simulink library "controllerComponents"  (R2018a)
settings: Solver=VariableStepAuto  StartTime=0.0  StopTime=10.0  RelTol=1e-3
undefined symbols (not defined in the file): p
libraries: simulink x2, dspsigops x1
settings Model: Creator=mitch  LastModifiedBy=mcobb

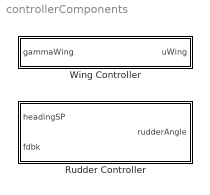
== system controllerComponents ==
  Rudder Controller : Subsystem
  Wing Controller : Subsystem

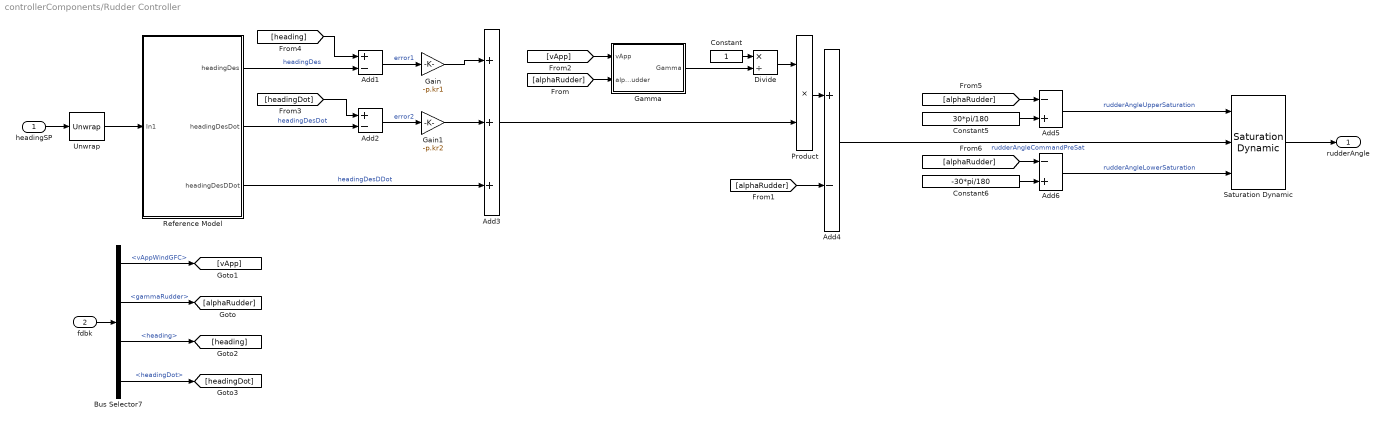
== system controllerComponents/Rudder Controller ==
  headingSP : Inport  Unit=rad
  fdbk : Inport  Port=2  OutDataTypeStr=Bus: busPlantFeedback
  Add1 : Sum  Inputs=+-
  Add2 : Sum  Inputs=+-
  Add3 : Sum  Inputs=+++
  Add4 : Sum  Inputs=+-
  Add5 : Sum  Inputs=-+
  Add6 : Sum  Inputs=-+
  Bus Selector7 : BusSelector  OutputSignals=vAppWindGFC,gammaRudder,heading,headingDot
  Constant : Constant
  Constant5 : Constant  Value=30*pi/180
  Constant6 : Constant  Value=-30*pi/180
  Divide : Product  Inputs=*/
  Gain : Gain  Gain=-p.kr1
  Gain1 : Gain  Gain=-p.kr2
  Gamma : Subsystem
  Product : Product
  Reference Model : Subsystem
  Saturation Dynamic : simulink/Discontinuities/Saturation Dynamic  OutMin=[]  OutMax=[]  OutDataTypeStr=Inherit: Same as second input  OutDataType=fixdt(1, 16)  OutScaling=2^-10  DoSatur=off
  Unwrap : dspsigops/Unwrap  tol=pi  InputProcessing=Columns as channels (frame based)  running=off
  rudderAngle : Outport  Unit=rad
  wires:
  [vApp] -> Gamma/1(vApp)
  [alphaRudder] -> Gamma/2(alphaRudder)
  [alphaRudder] -> Add4/2
  Product/1 -> Add4/1
  Gamma/1(Gamma) -> Divide/2
  Divide/1 -> Product/1
  Constant/1 -> Divide/1
  Add2/1 -> Gain1/1  "error2"
  Add1/1 -> Gain/1  "error1"
  Reference Model/1(headingDes) -> Add1/2  "headingDes"
  Reference Model/2(headingDesDot) -> Add2/2  "headingDesDot"
  [heading] -> Add1/1
  Gain1/1 -> Add3/2
  [headingDot] -> Add2/1
  Reference Model/3(headingDesDDot) -> Add3/3  "headingDesDDot"
  Gain/1 -> Add3/1
  Add3/1 -> Product/2
  fdbk/1 -> Bus Selector7/1
  Bus Selector7/4 -> [headingDot]  "<headingDot>"
  Bus Selector7/3 -> [heading]  "<heading>"
  Bus Selector7/2 -> [alphaRudder]  "<gammaRudder>"
  Bus Selector7/1 -> [vApp]  "<vAppWindGFC>"
  headingSP/1 -> Unwrap/1
  Unwrap/1 -> Reference Model/1(In1)
  Constant6/1 -> Add6/2
  Add4/1 -> Saturation Dynamic/2  "rudderAngleCommandPreSat"
  Saturation Dynamic/1 -> rudderAngle/1
  [alphaRudder] -> Add5/1
  Constant5/1 -> Add5/2
  Add5/1 -> Saturation Dynamic/1  "rudderAngleUpperSaturation"
  Add6/1 -> Saturation Dynamic/3  "rudderAngleLowerSaturation"
  [alphaRudder] -> Add6/1

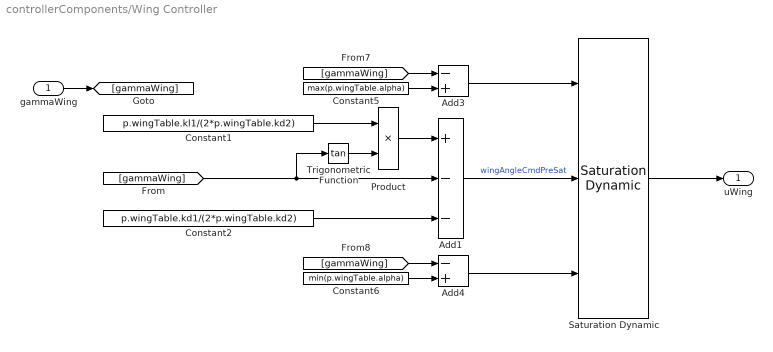
== system controllerComponents/Wing Controller ==
  gammaWing : Inport  Unit=rad
  Add1 : Sum  Inputs=+--
  Add3 : Sum  Inputs=-+
  Add4 : Sum  Inputs=-+
  Constant1 : Constant  Value=p.wingTable.kl1/(2*p.wingTable.kd2)
  Constant2 : Constant  Value=p.wingTable.kd1/(2*p.wingTable.kd2)
  Constant5 : Constant  Value=max(p.wingTable.alpha)
  Constant6 : Constant  Value=min(p.wingTable.alpha)
  Product : Product
  Saturation Dynamic : simulink/Discontinuities/Saturation Dynamic  OutMin=[]  OutMax=[]  OutDataTypeStr=Inherit: Same as second input  OutDataType=fixdt(1, 16)  OutScaling=2^-10  DoSatur=off
  Trigonometric Function : Trigonometry  Operator=tan
  uWing : Outport  Unit=rad
  wires:
  Trigonometric Function/1 -> Product/2
  Product/1 -> Add1/1
  Constant1/1 -> Product/1
  gammaWing/1 -> [gammaWing]
  [gammaWing] -> Add1/2, Trigonometric Function/1
  Add1/1 -> Saturation Dynamic/2  "wingAngleCmdPreSat"
  Saturation Dynamic/1 -> uWing/1
  [gammaWing] -> Add3/1
  Constant5/1 -> Add3/2
  Add3/1 -> Saturation Dynamic/1
  Constant6/1 -> Add4/2
  [gammaWing] -> Add4/1
  Add4/1 -> Saturation Dynamic/3
  Constant2/1 -> Add1/3

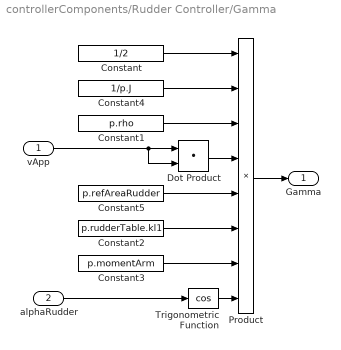
== system controllerComponents/Rudder Controller/Gamma ==
  vApp : Inport
  alphaRudder : Inport  Port=2
  Constant : Constant  Value=1/2
  Constant1 : Constant  Value=p.rho
  Constant2 : Constant  Value=p.rudderTable.kl1
  Constant3 : Constant  Value=p.momentArm
  Constant4 : Constant  Value=1/p.J
  Constant5 : Constant  Value=p.refAreaRudder
  Dot Product : DotProduct  InputSameDT=on  OutDataTypeStr=Inherit: Inherit via internal rule
  Product : Product  Inputs=8
  Trigonometric Function : Trigonometry  Operator=cos
  Gamma : Outport
  wires:
  Constant4/1 -> Product/2
  Constant3/1 -> Product/7
  Constant5/1 -> Product/5
  Constant/1 -> Product/1
  Constant2/1 -> Product/6
  Constant1/1 -> Product/3
  Dot Product/1 -> Product/4
  vApp/1 -> Dot Product/2, Dot Product/1
  alphaRudder/1 -> Trigonometric Function/1
  Trigonometric Function/1 -> Product/8
  Product/1 -> Gamma/1

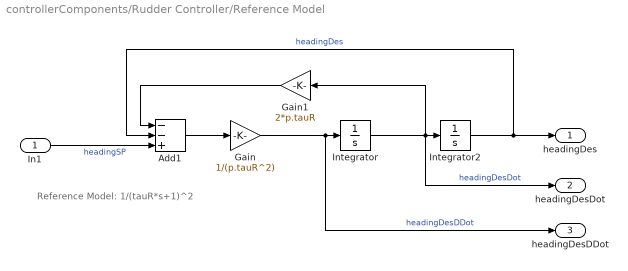
== system controllerComponents/Rudder Controller/Reference Model ==
  note: Reference Model:
      | 1/(tauR*s+1)^2
  In1 : Inport
  Add1 : Sum  Inputs=--+
  Gain : Gain  Gain=1/(p.tauR^2)
  Gain1 : Gain  Gain=2*p.tauR
  Integrator : Integrator
  Integrator2 : Integrator  InitialCondition=p.initTwist
  headingDes : Outport
  headingDesDot : Outport  Port=2
  headingDesDDot : Outport  Port=3
  wires:
  Gain/1 -> headingDesDDot/1, Integrator/1  "headingDesDDot"
  Integrator/1 -> headingDesDot/1, Gain1/1, Integrator2/1  "headingDesDot"
  Add1/1 -> Gain/1
  Integrator2/1 -> Add1/2, headingDes/1  "headingDes"
  In1/1 -> Add1/3  "headingSP"
  Gain1/1 -> Add1/1
